simulink model "tracking"  (Simulink 7.5)
settings: Solver=ode45  StartTime=0.0  StopTime=10.0  RelTol=1e-3
libraries: powerlib_extras x2, dspsigops x2, dspsrcs4 x2
settings Model: Creator=SISA  LastModifiedBy=SISA

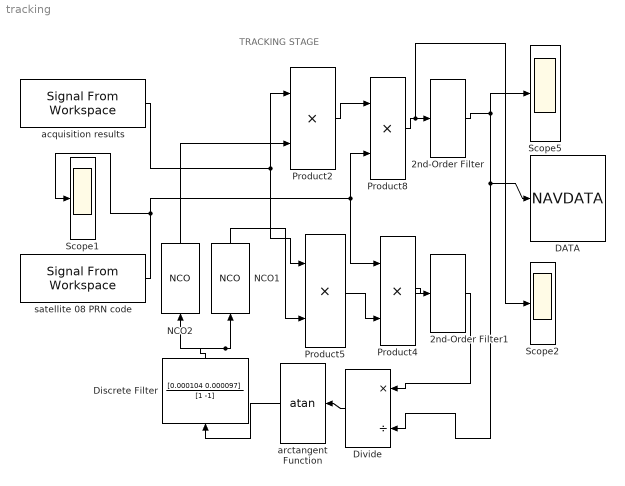
== system tracking ==
  note: TRACKING STAGE
  2nd-Order Filter : powerlib_extras/Control  Blocks/2nd-Order Filter  DialogController=POWERSYS.PowerSysDialog  SystemSampleTime=-1  FilterType=Lowpass  Fo=50  Zeta=0.707  Initialize=off  Vac_Init=[1 45 60]  Vdc_Init=-0.5  PlotResponse=off  param1=[1 500 1]
  2nd-Order Filter1 : powerlib_extras/Control  Blocks/2nd-Order Filter  DialogController=POWERSYS.PowerSysDialog  SystemSampleTime=-1  FilterType=Lowpass  Fo=50  Zeta=0.707  Initialize=off  Vac_Init=[1 45 60]  Vdc_Init=-0.5  PlotResponse=off  param1=[1 500 1]
  DATA : ToWorkspace  VariableName=NAVDATA  SampleTime=-1  SaveFormat=Array
      settings: MaxDataPoints=1023000
  Discrete Filter : DiscreteFilter  Numerator=[0.000104 0.000097]  Denominator=[1 -1]  SampleTime=1
  Divide : Product  Inputs=*/  OutDataType=fixdt(1, 16)  OutScaling=2^-10
  NCO1 : dspsigops/NCO  DialogController=dspdialog.NCO  AccIncSrc=Input port  AccInc=100  PhaseOffsetSrc=Specify via dialog  PhaseOffset=0  AccumWL=16  HasDither=on  DitherWL=4  PNgeneratorLength=19  HasPhaseQuantizer=on  TableDepth=12  HasOutputPhaseError=off  Formula=Sine  DataType=Binary point scaling  OutputWL=16  OutputFL=14  CompMethod=Table lookup (no interpolation)  SampleTime=1  SamplesPerFrame=1
  NCO2 : dspsigops/NCO  DialogController=dspdialog.NCO  AccIncSrc=Input port  AccInc=100  PhaseOffsetSrc=Specify via dialog  PhaseOffset=0  AccumWL=16  HasDither=on  DitherWL=4  PNgeneratorLength=19  HasPhaseQuantizer=on  TableDepth=12  HasOutputPhaseError=off  Formula=Cosine  DataType=Binary point scaling  OutputWL=16  OutputFL=14  CompMethod=Table lookup (no interpolation)  SampleTime=1  SamplesPerFrame=1
  Product{2,4..5,8} (4 alike) : Product  OutDataType=fixdt(1, 16)  OutScaling=2^0  RndMeth=Zero
  Scope1 : Scope
  Scope2 : Scope
      settings: SaveName=ScopeData2
  Scope5 : Scope
  acquisition results : dspsrcs4/Signal From Workspace  SystemSampleTime=-1  X=TRACK  Ts=1  nsamps=1  OutputAfterFinalValue=Setting to zero  ignoreOrWarnInputAndFrameLengths=off
  arctangent Function : Trigonometry  Operator=atan
  satellite 08 PRN code : dspsrcs4/Signal From Workspace  SystemSampleTime=-1  X=PN08  Ts=1  nsamps=1  OutputAfterFinalValue=Setting to zero  ignoreOrWarnInputAndFrameLengths=off
  wires:
  satellite 08 PRN code/1 -> Product8/2, Product4/1, Scope1/1
  NCO2/1 -> Product2/2
  Product4/1 -> 2nd-Order Filter1/1
  Product8/1 -> 2nd-Order Filter/1, Scope2/1
  Product2/1 -> Product8/1
  2nd-Order Filter1/1 -> Divide/1
  2nd-Order Filter/1 -> DATA/1, Divide/2, Scope5/1
  NCO1/1 -> Product5/2
  Discrete Filter/1 -> NCO1/1, NCO2/1
  Product5/1 -> Product4/2
  acquisition results/1 -> Product2/1, Product5/1
  Divide/1 -> arctangent Function/1
  arctangent Function/1 -> Discrete Filter/1
